simulink model "gpsModel01"  (R2023a)
settings: Solver=FixedStepDiscrete  StartTime=0.0  StopTime=480  RelTol=1e-3  EnableMultiTasking=on
libraries: sldrtlib x1
settings Model: SimulationMode=external  Creator=lion  LastModifiedBy=lion
settings SolverCC: AutoInsertRateTranBlk=on
settings DataIOCC: SaveOutput=off  SaveTime=off
settings OptimizationCC: DefaultParameterBehavior=Inlined  InlineInvariantSignals=on  EnhancedBackFolding=on  PassReuseOutputArgsThreshold=0  StateBitsets=on  DataBitsets=on  OptimizeBlockOrder=speed  DifferentSizesBufferReuse=on
settings DebuggingCC: ParameterTunabilityLossMsg=error
settings HardwareCC: ProdBitPerLong=64  ProdHWDeviceType=Intel->x86-64 (Linux 64)
settings SFSimCC: MATLABDynamicMemAlloc=off
settings RTWCC: Description=Simulink Desktop Real-Time  SystemTargetFile=sldrt.tlc  TLCOptions=-p0  TemplateMakefile=sldrt.tmf  GenerateReport=on  RTWVerbose=off  LaunchReport=on  RTWCompilerOptimization=on
settings CodeAppCC: ForceParamTrailComments=on  MaxIdLength=95  OperatorAnnotations=on
settings SimulinkDesktopRealTimeCC: TargetLibSuffix=_sldrt.a  TargetPreCompLibLocation=C:\Program Files\MATLAB\R2023a\toolbox\sldrt\lib\win64

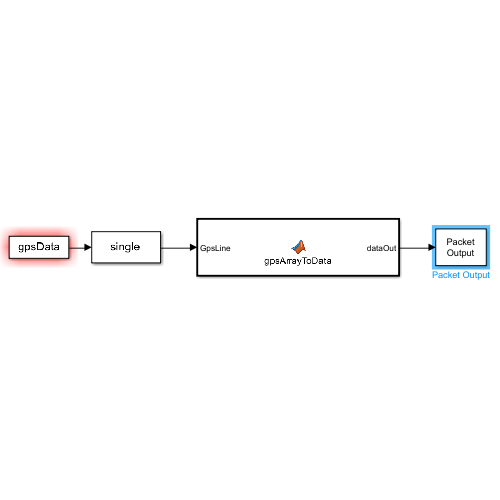
[thumbnail: Simulink's stored preview of the top-level diagram]
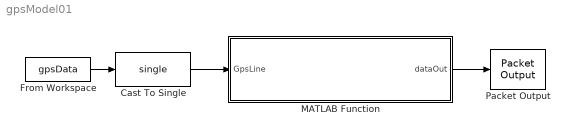
== system gpsModel01 ==
  Cast To Single : DataTypeConversion  OutDataTypeStr=single  SaturateOnIntegerOverflow=off  RndMeth=Floor
  From Workspace : FromWorkspace  VariableName=gpsData  OutDataTypeStr=double  SampleTime=1.0  OutputAfterFinalValue=Holding final value
  MATLAB Function : MATLAB Function  TreatAsAtomicUnit=on
  Packet Output : sldrtlib/Packet Output  SampleTime=0.1  MaxMissedTicks=10  ShowMissedTicks=off  YieldWhenWaiting=off  DrvAddress=0  DrvOptions=0  PacketSize=32  DataTypes='4*double'  ShowReady=off  ShowError=off  PacketID=1  ByteOrder=1  InitialValue=[]  FinalValue=[]
  wires:
  From Workspace/1 -> Cast To Single/1
  Cast To Single/1 -> MATLAB Function/1(GpsLine)
  MATLAB Function/1(dataOut) -> Packet Output/1

== matlab function gpsModel01/MATLAB Function ==
  data: GpsLine input; dataOut output
 function dataOut = gpsArrayToData(GpsLine)
dataOut = uint8(zeros(1, 56));
header = uint8([12,21,12,21]);
year = typecast(single(GpsLine(1)), 'uint8');
month = typecast(single(GpsLine(2)), 'uint8');
day = typecast(single(GpsLine(3)), 'uint8');
hour = typecast(single(GpsLine(4)), 'uint8');
minute = typecast(single(GpsLine(5)), 'uint8');
second = typecast(single(GpsLine(6)), 'uint8');
positionX = typecast(single(GpsLine(7)), 'uint8');
positionY = typecast(single(GpsLine(8)), 'uint8');
positionZ = typecast(single(GpsLine(9)), 'uint8');
velocityX = typecast(single(GpsLine(10)), 'uint8');
velocityY = typecast(single(GpsLine(11)), 'uint8');
velocityZ = typecast(single(GpsLine(12)), 'uint8');
checkSum = uint8([0,0,0,0]);
dataOut = [header, year, month, day, hour, minute, second, positionX, ...
    positionY, positionZ, velocityX, velocityY, velocityZ, checkSum];
end
